simulink model "Exp5Star"  (R2026a)
settings: Solver=VariableStepAuto
libraries: fl_lib x15, nesl_utility x5, eeRmsMeasurement x4

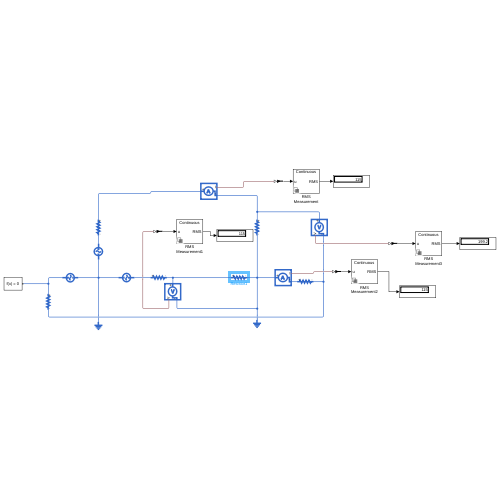
[thumbnail: Simulink's stored preview of the top-level diagram]
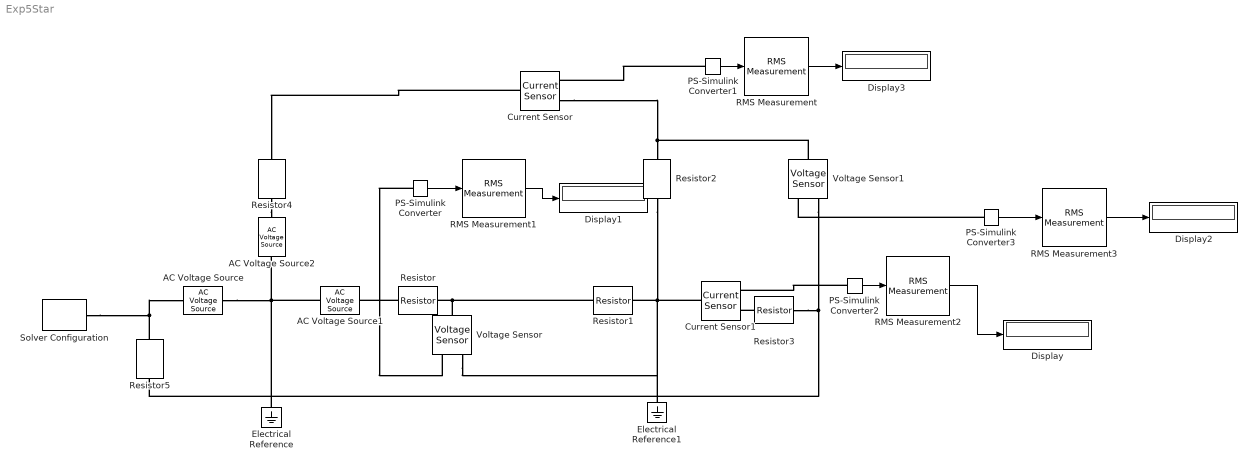
== system Exp5Star ==
  AC Voltage Source : fl_lib/Electrical/Electrical Sources/AC Voltage Source  amp=325.27 V  shift=-120 deg  frequency=50 Hz
  AC Voltage Source1 : fl_lib/Electrical/Electrical Sources/AC Voltage Source  amp=325.27 V  shift=120 deg  frequency=50 Hz
  AC Voltage Source2 : fl_lib/Electrical/Electrical Sources/AC Voltage Source  amp=325.27 V  shift=0 deg  frequency=50 Hz
  Current Sensor : fl_lib/Electrical/Electrical Sensors/Current Sensor
  Current Sensor1 : fl_lib/Electrical/Electrical Sensors/Current Sensor
  Display{,1..3} (4 alike) : Display
  Electrical Reference : fl_lib/Electrical/Electrical Elements/Electrical Reference
  Electrical Reference1 : fl_lib/Electrical/Electrical Elements/Electrical Reference
  PS-Simulink Converter{,1..3} (4 alike) : nesl_utility/PS-Simulink Converter  PhysicalDomain=network_engine_domain  SubClassName=ps_output  LeftPortType=input  RightPortType=output  PseudoPeriodic=off  Frequencies=[]  VectorFormat=inherit  Unit=inherit  AffineConversion=off
  RMS Measurement{,1..3} (4 alike) : eeRmsMeasurement/RMS Measurement  LabelModeActiveChoice=Total  F=50  SpecifyHarmonics=off  K=[0 1 2]  Ts=0
      settings: LibrarySourceBlock=|
      | ee_sl_lib/Measurements/RMS
      | Measurement
  Resistor{,1..5} (6 alike) : fl_lib/Electrical/Electrical Elements/Resistor  R=1 Ohm  i_specify=off  i_priority=None  i=0 A  i_nominal_specify=off  i_nominal_value=1  i_nominal_unit=A  v_specify=off  v_priority=None  v=0 V  v_nominal_specify=off  v_nominal_value=1  v_nominal_unit=V
  Solver Configuration : nesl_utility/Solver Configuration  PhysicalDomain=network_engine_domain  SubClassName=solver  LeftPortType=input  RightPortType=generic  Tones=[]  Harmonics=[]  SimulateNoise=off  Profile=off  UseLocalSampling=off  EnableSwitchedLinearOptims=on  FrequencyDomain=off  UseCCode=off  RelTol=0.001  AbsTol=0.001  MinStep=1e-09  ToWorkspace=off  RevertToSquareIcSolve=off  NumHomotopyIterations=100  PhasorMode=off  PhasorModeNumHarmonics=1  ConsistencySolver=NEWTON_XTOL_AFTER_FTOL  CanonicalOrdering=CANONICAL  OptimizeIntermediates=OPTIMIZED  IndexReductionMethod=DerivativeReplacement  DoDC=off  ResidualTolerance=1e-09  ConsistencyTolSource=GLOBAL  ConsistencyAbsTol=0.001  ConsistencyRelTol=0.001  ConsistencyTolFactor=0.001  UseLocalSolver=off  LocalSolverChoice=NE_BACKWARD_EULER_ADVANCER  ResolveIndetEquations=on  FunctionEvalNumThread=1  LocalSolverSampleTime=0.001  DoFixedCost=off  MaxNonlinIter=3  MaxModeIter=2  ComputeImpulses=off  ImpulseIterations=2  LinearAlgebra=auto  LinearAlgebraNumThread=0  EquationFormulation=NE_TIME_EF  DelaysMemoryBudget=1024  AutomaticFiltering=on  FilteringTimeConstant=0.001  PartitionStorageMethod=AS_NEEDED  PartitionMemoryBudget=1024  PartitionMethod=ROBUST  MultibodyUseLocalSolver=off  MultibodyLocalSolverChoice=ODE1  MultibodyLocalSolverSampleTime=0.001
  Voltage Sensor : fl_lib/Electrical/Electrical Sensors/Voltage Sensor
  Voltage Sensor1 : fl_lib/Electrical/Electrical Sensors/Voltage Sensor
  wires:
  PS-Simulink Converter1/1 -> RMS Measurement/1
  RMS Measurement/1 -> Display3/1
  PS-Simulink Converter/1 -> RMS Measurement1/1
  PS-Simulink Converter2/1 -> RMS Measurement2/1
  RMS Measurement2/1 -> Display/1
  PS-Simulink Converter3/1 -> RMS Measurement3/1
  RMS Measurement3/1 -> Display2/1
  RMS Measurement1/1 -> Display1/1
  connections:
  Resistor4/RConn1 -- AC Voltage Source2/LConn1
  Resistor5/LConn1 -- AC Voltage Source/LConn1 -- Solver Configuration/RConn1
  Resistor/LConn1 -- AC Voltage Source1/LConn1
  Electrical Reference/LConn1 -- AC Voltage Source/RConn1 -- AC Voltage Source1/RConn1 -- AC Voltage Source2/RConn1
  PS-Simulink Converter1/LConn1 -- Current Sensor/RConn1
  PS-Simulink Converter/LConn1 -- Voltage Sensor/RConn1
  PS-Simulink Converter2/LConn1 -- Current Sensor1/RConn1
  PS-Simulink Converter3/LConn1 -- Voltage Sensor1/RConn1
  Resistor1/LConn1 -- Voltage Sensor/LConn1 -- Resistor/RConn1
  Resistor2/RConn1 -- Voltage Sensor/RConn2 -- Electrical Reference1/LConn1 -- Current Sensor1/LConn1 -- Resistor1/RConn1
  Resistor3/LConn1 -- Current Sensor1/RConn2
  Resistor3/RConn1 -- Voltage Sensor1/RConn2 -- Resistor5/RConn1
  Current Sensor/LConn1 -- Resistor4/LConn1
  Current Sensor/RConn2 -- Voltage Sensor1/LConn1 -- Resistor2/LConn1
